simulink model "HILController_sim"  (R2017a)
settings: Solver=FixedStepAuto  StartTime=0.0  StopTime=Endtime  FixedStep=0.05  RelTol=1e-3  EnableMultiTasking=on
values from neighbouring files (symbols this model uses):
  kc = 0.0273    [HILS_Controller_Setting.m]
  SV = 1000    [HILS_Controller_Setting.m]
  Td = 0    [HILS_Controller_Setting.m]
  Ti = 18.2    [HILS_Controller_Setting.m]
libraries: arduinolib x6
settings Model: SimulationMode=external  ExtModeTrigDuration=2  Creator=Shin  LastModifiedBy=SHRUTI
settings OptimizationCC: LifeSpan=Inf  MaxStackSize=64
settings DebuggingCC: SFUnexpectedBacktrackingDiag=warning  SFNoUnconditionalDefaultTransitionDiag=warning  SFExecutionAtInitializationDiag=none
settings HardwareCC: ProdBitPerInt=16  ProdBitPerPointer=16  ProdBitPerSizeT=16  ProdBitPerPtrDiffT=16  ProdLargestAtomicFloat=None  ProdWordSize=8  ProdHWDeviceType=Atmel->AVR  UseEmbeddedCoderFeatures=off  UseSimulinkCoderFeatures=off
settings RTWCC: SystemTargetFile=ert.tlc  HardwareBoard=Arduino Mega 2560  TLCOptions=-aInlineSetEventsForThisBaseRateFcn=TLC_FALSE -aSuppressMultiTaskScheduler=TLC_FALSE -aRateBasedStepFcn=1  TemplateMakefile=ert_default_tmf  Description=Embedded Coder  GenerateReport=on  Toolchain=Arduino AVR  BuildConfiguration=Faster Runs  LaunchReport=on
settings CodeAppCC: ForceParamTrailComments=on  OperatorAnnotations=on  MATLABSourceComments=on
settings ERTTargetCC: MultiwordLength=2048  ERTCustomFileBanners=off  SupportContinuousTime=on  SupportNonInlinedSFcns=on  RemoveResetFunc=off  SupportVariableSizeSignals=on  ModelStepFunctionPrototypeControlCompliant=off
settings ConfigComp: CovMetricSettings=dw  CovHtmlReporting=on  CovSaveCumulativeToWorkspaceVar=on  CovSaveSingleToWorkspaceVar=on  CovExternalEMLEnable=off

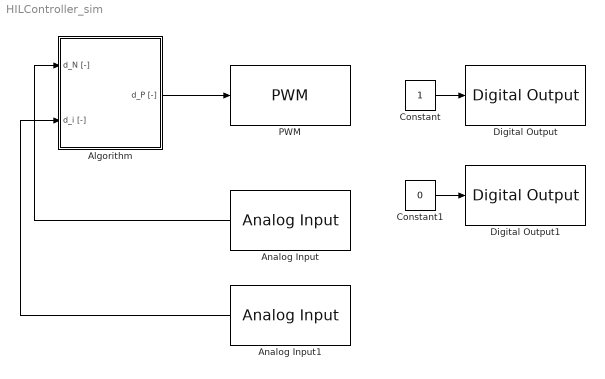
== system HILController_sim ==
  Algorithm : Subsystem
  Analog Input : arduinolib/Analog Input  pinNumber=5  sampleTime=0  blockPlatform=arduino
  Analog Input1 : arduinolib/Analog Input  pinNumber=6  sampleTime=0  blockPlatform=arduino
  Constant : Constant
  Constant1 : Constant  Value=0
  Digital Output : arduinolib/Digital Output  pinNumber=7  blockPlatform=arduino
  Digital Output1 : arduinolib/Digital Output  pinNumber=8  blockPlatform=arduino
  PWM : arduinolib/PWM  pinNumber=10  blockPlatform=arduino
  wires:
  Algorithm/1(d_P [-]) -> PWM/1
  Analog Input/1 -> Algorithm/1(d_N [-])
  Analog Input1/1 -> Algorithm/2(d_i [-])
  Constant/1 -> Digital Output/1
  Constant1/1 -> Digital Output1/1

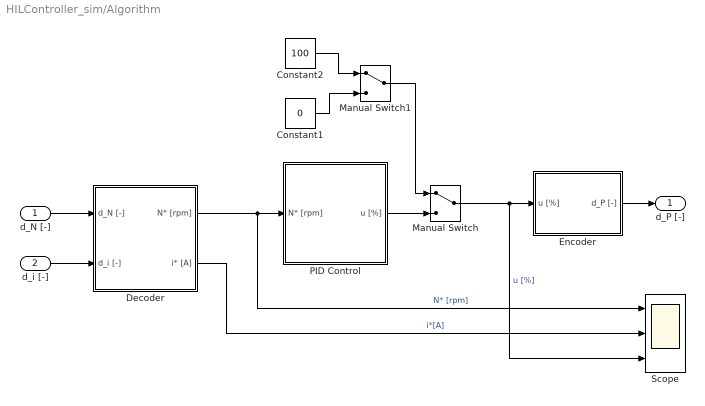
== system HILController_sim/Algorithm ==
  d_N [-] : Inport
  d_i [-] : Inport  Port=2
  Constant1 : Constant  Value=0
  Constant2 : Constant  Value=100
  Decoder : Subsystem
  Encoder : Subsystem
  Manual Switch : ManualSwitch
  Manual Switch1 : ManualSwitch
  PID Control : Subsystem
  Scope : Scope  NumInputPorts=3
  d_P [-] : Outport
  wires:
  d_N [-]/1 -> Decoder/1(d_N [-])
  Encoder/1(d_P [-]) -> d_P [-]/1
  Decoder/1(N* [rpm]) -> Scope/1, PID Control/1(N* [rpm])  "N* [rpm]"
  d_i [-]/1 -> Decoder/2(d_i [-])
  Manual Switch/1 -> Scope/3, Encoder/1(u [%])  "u [%]"
  PID Control/1(u [%]) -> Manual Switch/2
  Manual Switch1/1 -> Manual Switch/1
  Constant2/1 -> Manual Switch1/1
  Constant1/1 -> Manual Switch1/2
  Decoder/2(i* [A]) -> Scope/2  "i*[A]"

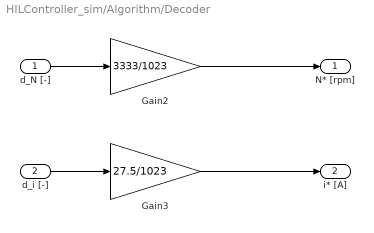
== system HILController_sim/Algorithm/Decoder ==
  d_N [-] : Inport
  d_i [-] : Inport  Port=2
  Gain2 : Gain  Gain=3333/1023
  Gain3 : Gain  Gain=27.5/1023
  N* [rpm] : Outport
  i* [A] : Outport  Port=2
  wires:
  Gain2/1 -> N* [rpm]/1
  d_N [-]/1 -> Gain2/1
  Gain3/1 -> i* [A]/1
  d_i [-]/1 -> Gain3/1

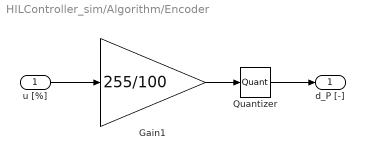
== system HILController_sim/Algorithm/Encoder ==
  u [%] : Inport
  Gain1 : Gain  Gain=255/100
  Quantizer : Quantizer
  d_P [-] : Outport
  wires:
  Gain1/1 -> Quantizer/1
  u [%]/1 -> Gain1/1
  Quantizer/1 -> d_P [-]/1

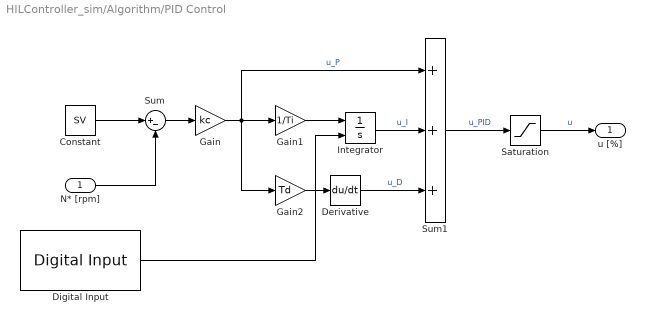
== system HILController_sim/Algorithm/PID Control ==
  N* [rpm] : Inport
  Constant : Constant  Value=SV
  Derivative : Derivative
  Digital Input : arduinolib/Digital Input  pinNumber=3  sampleTime=0  blockPlatform=arduino
      settings: SourceProductName=Simulink Support Package for Arduino Hardware
  Gain : Gain  Gain=kc
  Gain1 : Gain  Gain=1/Ti
  Gain2 : Gain  Gain=Td
  Integrator : Integrator  ExternalReset=falling
  Saturation : Saturate  UpperLimit=100  LowerLimit=0
  Sum : Sum  Inputs=|+-
  Sum1 : Sum  Inputs=+++
  u [%] : Outport
  wires:
  N* [rpm]/1 -> Sum/2
  Constant/1 -> Sum/1
  Sum1/1 -> Saturation/1  "u_PID"
  Sum/1 -> Gain/1
  Gain/1 -> Sum1/1, Gain1/1, Gain2/1  "u_P"
  Gain1/1 -> Integrator/1
  Gain2/1 -> Derivative/1
  Derivative/1 -> Sum1/3  "u_D"
  Integrator/1 -> Sum1/2  "u_I"
  Saturation/1 -> u [%]/1  "u"
  Digital Input/1 -> Integrator/2
